simulink model "pitchRate_controller_simulink"  (R2024b)
settings: Solver=VariableStepAuto  StartTime=0.0  StopTime=10  RelTol=1e-3
values from neighbouring files (symbols this model uses):
  A_ac_p4 = A_long_p4([1,2],[1,2])    [HA_ES_MainCode.m]    (also in PitchController.mat = [-0.526053716536  0.926966812108; -1.23331740816  -0.7913865)
  B_ac_p4 = A_long_p4([1,2],3)    [HA_ES_MainCode.m]    (also in PitchController.mat = [-0.00111817696757 -0.0656846818337])
  C_ac_p4 = C_long_p4([1,2],[1,2])    [HA_ES_MainCode.m]    (also in PitchController.mat = [57.2957795131  0; 0  57.2957795131])
  D_ac_p4 = C_long_p4([1,2],3)    [HA_ES_MainCode.m]    (also in PitchController.mat = [0 0])
  s = tf("s")    [HA_ES_MainCode.m]
libraries: slctrl_linear x1
settings Model: PacingRate=0.100000  Creator=henryadam  LastModifiedBy=henryadam

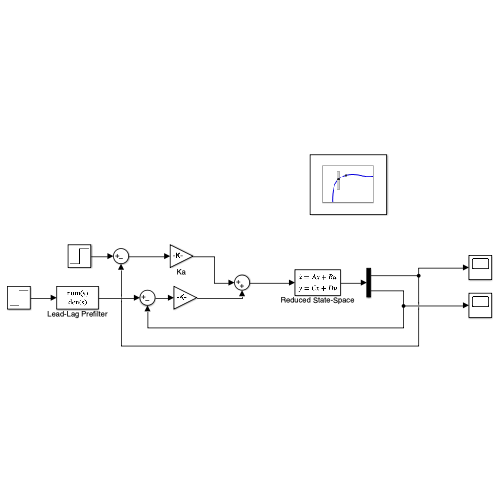
[thumbnail: Simulink's stored preview of the top-level diagram]
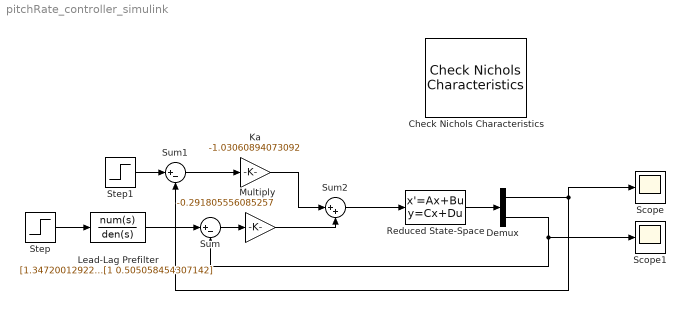
== system pitchRate_controller_simulink ==
  Check Nichols Characteristics : slctrl_linear/Check Nichols Characteristics  InstantiateOnLoad=on  SaveOperatingPoints=off  LinearizationIOs={'/Demux', 2, 'out', 'off', '';'/Sum2', 1, 'in', 'on', ''}  LinearizeAt=SnapshotTimes  SnapshotTimes=[0]  TriggerType=rising  SampleTime=auto  RateConversionMethod=zoh  PreWarpFreq=10  UseExactDelayModel=off  UseFullBlockNameLabels=off  UseBusSignalLabels=off  enabled=on  stopWhenAssertionFail=off  export=off  ViewDlgPos=[368 148 725 621]  LaunchViewOnOpen=off  OpenViewOnLoad=off  FrequencyUnits=rad/s  MagnitudeUnits=dB  PhaseUnits=deg  TimeUnits=seconds  EnableMargins=on  GainMargin=20  PhaseMargin=30  EnableGainPhaseBound=off  GainPhaseBoundType={'upper'}  OLPhases=[]  OLGains=[]  EnableCLPeakGain=off  CLPeakGain=[]  FeedbackSign=-1
      settings: SaveToWorkspace=off  SaveName=sys
      settings: LibrarySourceBlock=|
      | slctrlblks/Model Verification/Check Nichols
      | Characteristics
  Demux : Demux  Outputs=2
  Ka : Gain  Gain=-1.03060894073092
  Lead-Lag Prefilter : TransferFcn  Numerator=[1.3472001292297e-12 5.24663894955974]  Denominator=[1 0.505058454307142]
  Multiply : Gain  Gain=-0.291805556085257
  Reduced State-Space : StateSpace  A=A_ac_p4  B=B_ac_p4  C=C_ac_p4  D=D_ac_p4  InitialCondition=0
  Scope : Scope
  Scope1 : Scope
  Step : Step  SampleTime=0
  Step1 : Step  After=0  SampleTime=0
  Sum : Sum  Inputs=|+-
  Sum1 : Sum  Inputs=|+-
  Sum2 : Sum  Inputs=|++
  wires:
  Reduced State-Space/1 -> Demux/1
  Step1/1 -> Sum1/1
  Sum1/1 -> Ka/1
  Demux/2 -> Sum/2, Scope1/1
  Demux/1 -> Scope/1, Sum1/2
  Ka/1 -> Sum2/1
  Multiply/1 -> Sum2/2
  Sum2/1 -> Reduced State-Space/1
  Sum/1 -> Multiply/1
  Step/1 -> Lead-Lag Prefilter/1
  Lead-Lag Prefilter/1 -> Sum/1
